simulink model "park_examen"  (R2017b)
settings: Solver=VariableStepAuto  StartTime=0.0  StopTime=0.08  MaxStep=1e-4  RelTol=1e-3
values from neighbouring files (symbols this model uses):
  F_b = 50.0    (= 50)    [pll_phasor.m]
undefined symbols (not defined in the file or in its folder): L, R, T_s_power
libraries: powerlib x6, powerlib_meascontrol x3
settings Model: Creator=jmmauricio  LastModifiedBy=jmmau
settings CodeAppCC: StateflowObjectComments=on
settings SimscapeCC: SimscapeNormalizeSystem=off

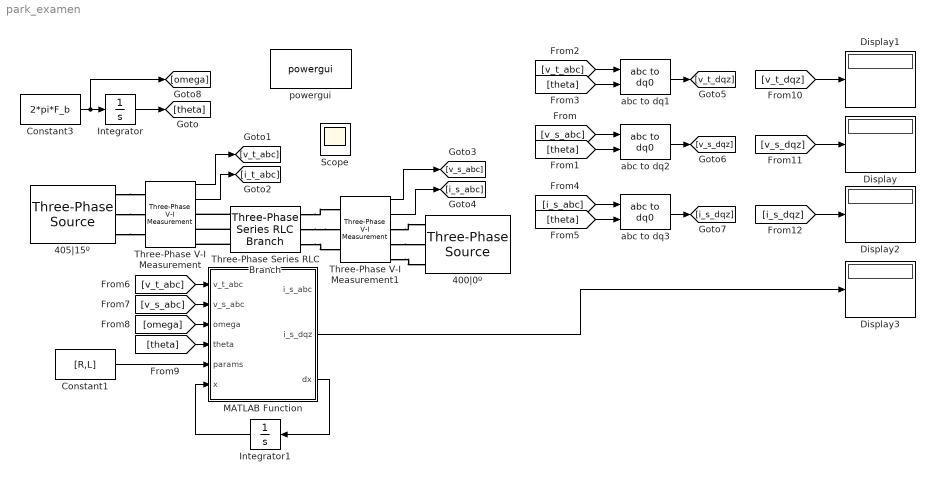
== system park_examen ==
  400|0º : powerlib/Electrical Sources/Three-Phase Source  InternalConnection=Yg  VoltagePhases=off  Voltage=400  PhaseAngle=0  Voltage_phases=[25e3 25e3 25e3]/sqrt(3)  PhaseAngles_phases=[0 -120 +120]  Frequency=50  NonIdealSource=on  SpecifyImpedance=off  Resistance=0.8929  Inductance=16.58e-3  ShortCircuitLevel=100e6  BaseVoltage=25e3  XRratio=7  BusType=swing  Pref=10e3  Qref=0  Prefabc=[10e3, 10e3, 10e3]  Qrefabc=[0, 0, 0]  Qmin=-inf  Qmax=inf
  405|15º : powerlib/Electrical Sources/Three-Phase Source  InternalConnection=Yg  VoltagePhases=off  Voltage=405  PhaseAngle=15  Voltage_phases=[25e3 25e3 25e3]/sqrt(3)  PhaseAngles_phases=[0 -120 +120]  Frequency=50  NonIdealSource=on  SpecifyImpedance=off  Resistance=0.8929  Inductance=16.58e-3  ShortCircuitLevel=100e6  BaseVoltage=25e3  XRratio=7  BusType=swing  Pref=10e3  Qref=0  Prefabc=[10e3, 10e3, 10e3]  Qrefabc=[0, 0, 0]  Qmin=-inf  Qmax=inf
  Constant1 : Constant  Value=[R,L]
  Constant3 : Constant  Value=2*pi*F_b
  Display{,1..3} (4 alike) : Display
  Integrator : Integrator
  Integrator1 : Integrator  InitialCondition=[0,0]
  MATLAB Function : MATLAB Function  TreatAsAtomicUnit=on
  Scope : Scope
  Three-Phase Series RLC Branch : powerlib/Elements/Three-Phase Series RLC Branch  LConnTagsString=A|B|C  RConnTagsString=A|B|C  BranchType=RL  Resistance=R  Inductance=L  Capacitance=1e-6  Measurements=None
  Three-Phase V-I Measurement : powerlib/Measurements/Three-Phase V-I Measurement  VoltageMeasurement=phase-to-ground  SetLabelV=off  LabelV=Vabc  Vpu=off  VpuLL=off  CurrentMeasurement=yes  SetLabelI=off  LabelI=Iabc  Ipu=off  Pbase=100e6  Vbase=500e3  OutputType=Complex  PhasorSimulation=off  PSBequivalent=0
  Three-Phase V-I Measurement1 : powerlib/Measurements/Three-Phase V-I Measurement  VoltageMeasurement=phase-to-ground  SetLabelV=off  LabelV=Vabc  Vpu=off  VpuLL=off  CurrentMeasurement=yes  SetLabelI=off  LabelI=Iabc  Ipu=off  Pbase=100e6  Vbase=500e3  OutputType=Complex  PhasorSimulation=off  PSBequivalent=0
  abc to dq1 : powerlib_meascontrol/Transformations/abc to dq0  Alignment=Aligned with phase A axis
  abc to dq2 : powerlib_meascontrol/Transformations/abc to dq0  Alignment=Aligned with phase A axis
  abc to dq3 : powerlib_meascontrol/Transformations/abc to dq0  Alignment=Aligned with phase A axis
  powergui : powerlib/powergui  Priority=1  SimulationMode=Continuous  SampleTime=T_s_power  frequency=60  Iterations=50  frequencyindice=50  Pbase=100e6  ErrMax=1e-4  UnitsV=kV  UnitsW=MW  buscounter=0  FunctionMessages=off  echomessages=off  EnableUseOfTLC=off  CurrentSourceSwitches=off  DisableSnubberDevices=off  DisableRonSwitches=off  DisableVfSwitches=off  DisplayEquations=off  SolverType=Tustin/Backward Euler (TBE)  Interpol=off  ExternalGateDelay=off  methode=off  Ts=100  x0status=blocks  SPID=on  SwTol=0  HookPort=off  RestoreLinks=warning  ResistiveCurrentMeasurement=off  Frange=[0:2:500]  Ylog=off  Xlog=on  ShowGrid=off  save=off  variable=ZData  structure=0  ZoomFFT=off  StartTime=0.0  cycles=1  DisplayStyle=1  fundamental=60  FreqAxis=off  MaxFrequency=1000  frequencyindicesteady=1  RmsSteady=1  display=off
  wires:
  Constant3/1 -> [omega], Integrator/1
  Integrator/1 -> [theta]
  Three-Phase V-I Measurement/1 -> [v_t_abc]
  Three-Phase V-I Measurement/2 -> [i_t_abc]
  Three-Phase V-I Measurement1/2 -> [i_s_abc]
  Three-Phase V-I Measurement1/1 -> [v_s_abc]
  [v_s_abc] -> abc to dq2/1
  [theta] -> abc to dq2/2
  [v_t_abc] -> abc to dq1/1
  [theta] -> abc to dq1/2
  [i_s_abc] -> abc to dq3/1
  [theta] -> abc to dq3/2
  abc to dq1/1 -> [v_t_dqz]
  abc to dq2/1 -> [v_s_dqz]
  abc to dq3/1 -> [i_s_dqz]
  [v_t_abc] -> MATLAB Function/1(v_t_abc)
  [v_s_abc] -> MATLAB Function/2(v_s_abc)
  [omega] -> MATLAB Function/3(omega)
  [theta] -> MATLAB Function/4(theta)
  Constant1/1 -> MATLAB Function/5(params)
  Integrator1/1 -> MATLAB Function/6(x)
  MATLAB Function/3(dx) -> Integrator1/1
  [v_t_dqz] -> Display1/1
  [v_s_dqz] -> Display/1
  [i_s_dqz] -> Display2/1
  MATLAB Function/2(i_s_dqz) -> Display3/1
  connections:
  405|15º/RConn1 -- Three-Phase V-I Measurement/LConn1
  405|15º/RConn2 -- Three-Phase V-I Measurement/LConn2
  405|15º/RConn3 -- Three-Phase V-I Measurement/LConn3
  Three-Phase Series RLC Branch/LConn1 -- Three-Phase V-I Measurement/RConn1
  Three-Phase Series RLC Branch/LConn2 -- Three-Phase V-I Measurement/RConn2
  Three-Phase Series RLC Branch/LConn3 -- Three-Phase V-I Measurement/RConn3
  Three-Phase V-I Measurement1/RConn3 -- 400|0º/RConn3
  Three-Phase V-I Measurement1/RConn2 -- 400|0º/RConn2
  Three-Phase V-I Measurement1/RConn1 -- 400|0º/RConn1
  Three-Phase Series RLC Branch/RConn1 -- Three-Phase V-I Measurement1/LConn1
  Three-Phase Series RLC Branch/RConn2 -- Three-Phase V-I Measurement1/LConn2
  Three-Phase Series RLC Branch/RConn3 -- Three-Phase V-I Measurement1/LConn3

== matlab function park_examen/MATLAB Function ==
  data: v_t_abc input; i_s_abc output; i_s_dqz output; v_s_abc input; omega input; theta input; params input; x input; dx output
function [i_s_abc,i_s_dqz,dx] = fcn(v_t_abc,v_s_abc,omega,theta,params,x)

R = params(1);
L = params(2);

T_p = 2.0/3.0*[[ cos(theta), cos(theta-2.0/3.0*pi), cos(theta+2.0/3.0*pi)],
               [-sin(theta),-sin(theta-2.0/3.0*pi),-sin(theta+2.0/3.0*pi)],
               [        0.5,                   0.5,                   0.5]];
           

T_p_inv = [[            cos(theta),            -sin(theta), 1.0],
           [ cos(theta-2.0/3.0*pi), -sin(theta-2.0/3.0*pi), 1.0],
           [ cos(theta+2.0/3.0*pi), -sin(theta+2.0/3.0*pi), 1.0]];

v_t_dqz = T_p * v_t_abc;
v_s_dqz = T_p * v_s_abc;

i_s_d = x(1);
i_s_q = x(2);

di_s_d = 1/L*(v_t_d - R*i_s_d - L*omega*i_s_q - v_s_d);
di_s_q = 1/L*(v_t_q - R*i_s_q - L*omega*i_s_d - v_s_q);

i_s_dqz = [i_s_d,i_s_q,0].';

i_s_abc = T_p * i_s_dqz;

dx = [di_s_d; di_s_q];
